simulink model "SWC_FDC_type"  (R2021b)
settings: Solver=FixedStepDiscrete  StartTime=0.0  StopTime=10.0  FixedStep=0.001  RelTol=1e-3
values from neighbouring files (symbols this model uses):
  DID_VCUKey = uint16(0x0202)    [vcu_local_hdr.m]
  DID_XWD = uint16(513)    [vcu_local_hdr.m]
  DIDLen_APSFunConfig = uint16(16)    [vcu_local_hdr.m]
  DIDLen_AutoLock = uint16(1)    [vcu_local_hdr.m]
  DIDLen_DKCKey = uint16(8)    [vcu_local_hdr.m]
  DIDLen_DRLDis = uint16(1)    [vcu_local_hdr.m]
  DIDLen_DynoMode = uint16(1)    [vcu_local_hdr.m]
  DIDLen_FMHTimer = uint16(1)    [vcu_local_hdr.m]
  DIDLen_LFLowPresThre = uint16(1)    [vcu_local_hdr.m]
  DIDLen_LFSensorID = uint16(4)    [vcu_local_hdr.m]
  DIDLen_LRLowPresThre = uint16(1)    [vcu_local_hdr.m]
  DIDLen_LRSensorID = uint16(4)    [vcu_local_hdr.m]
  DIDLen_RFLowPresThre = uint16(1)    [vcu_local_hdr.m]
  DIDLen_RFSensorID = uint16(4)    [vcu_local_hdr.m]
  DIDLen_RRLowPresThre = uint16(1)    [vcu_local_hdr.m]
  DIDLen_RRSensorID = uint16(4)    [vcu_local_hdr.m]
  DIDLen_SensorMode = uint16(1)    [vcu_local_hdr.m]
  DIDLen_TireSize = uint16(16)    [vcu_local_hdr.m]
  DIDLen_TPMSLearnSta = uint16(1)    [vcu_local_hdr.m]
  DIDLen_TurnLampFLThreCurr = uint16(1)    [vcu_local_hdr.m]
  DIDLen_TurnLampFRThreCurr = uint16(1)    [vcu_local_hdr.m]
  DIDLen_TurnLampRLThreCurr = uint16(1)    [vcu_local_hdr.m]
  DIDLen_TurnLampRRThreCurr = uint16(1)    [vcu_local_hdr.m]
  DIDLen_USSConfig = uint16(16)    [vcu_local_hdr.m]
  DIDLen_WhlPres = uint16(4)    [vcu_local_hdr.m]
  DIDLen_WhlSensorBattSta = uint16(1)    [vcu_local_hdr.m]
  DIDLen_WhlTmp = uint16(4)    [vcu_local_hdr.m]
  DIDLen_XWDMode = uint16(1)    [vcu_local_hdr.m]
  DIDNum_APSFunConfig = uint16(0x0903)    [vcu_local_hdr.m]
  DIDNum_AutoLock = uint16(0x0306)    [vcu_local_hdr.m]
  DIDNum_DKCKey = uint16(0x0202)    [vcu_local_hdr.m]
  DIDNum_DRLDis = uint16(0x0307)    [vcu_local_hdr.m]
  DIDNum_DynoMode = uint16(0x0203)    [vcu_local_hdr.m]
  DIDNum_FMHTimer = uint16(0x0305)    [vcu_local_hdr.m]
  DIDNum_LFLowPresThre = uint16(0x0B08)    [vcu_local_hdr.m]
  DIDNum_LFSensorID = uint16(0x0B01)    [vcu_local_hdr.m]
  DIDNum_LRLowPresThre = uint16(0x0B0A)    [vcu_local_hdr.m]
  DIDNum_LRSensorID = uint16(0x0B03)    [vcu_local_hdr.m]
  DIDNum_RFLowPresThre = uint16(0x0B09)    [vcu_local_hdr.m]
  DIDNum_RFSensorID = uint16(0x0B02)    [vcu_local_hdr.m]
  DIDNum_RRLowPresThre = uint16(0x0B0B)    [vcu_local_hdr.m]
  DIDNum_RRSensorID = uint16(0x0B04)    [vcu_local_hdr.m]
  DIDNum_SensorMode = uint16(0x0B0C)    [vcu_local_hdr.m]
  DIDNum_TireSize = uint16(0x0902)    [vcu_local_hdr.m]
  DIDNum_TPMSLearnSta = uint16(0x0B0D)    [vcu_local_hdr.m]
  DIDNum_TurnLampFLThreCurr = uint16(0x0303)    [vcu_local_hdr.m]
  DIDNum_TurnLampFRThreCurr = uint16(0x0301)    [vcu_local_hdr.m]
  DIDNum_TurnLampRLThreCurr = uint16(0x0304)    [vcu_local_hdr.m]
  DIDNum_TurnLampRRThreCurr = uint16(0x0302)    [vcu_local_hdr.m]
  DIDNum_USSConfig = uint16(0x0901)    [vcu_local_hdr.m]
  DIDNum_WhlPres = uint16(0x0B05)    [vcu_local_hdr.m]
  DIDNum_WhlSensorBattSta = uint16(0x0B07)    [vcu_local_hdr.m]
  DIDNum_WhlTmp = uint16(0x0B06)    [vcu_local_hdr.m]
  DIDNum_XWDMode = uint16(0x0201)    [vcu_local_hdr.m]
  DIDVCUKeyLength = uint16(8)    [vcu_local_hdr.m]
  ENUM_DRIVETRAIN_AWD = uint8(  2  )    [vcu_local_hdr.m]
  ENUM_DRIVETRAIN_FWD = uint8(  1  )    [vcu_local_hdr.m]
  ENUM_DRIVETRAIN_RWD = uint8(  0  )    [vcu_local_hdr.m]
  ENUM_REGENLEVEL_INVALID = uint8(  7  )    [vcu_local_hdr.m]
  ENUM_REGENLEVEL_LV1 = uint8(  1  )    [vcu_local_hdr.m]
  ENUM_REGENLEVEL_LV2 = uint8(  2  )    [vcu_local_hdr.m]
  ENUM_REGENLEVEL_LV3 = uint8(  3  )    [vcu_local_hdr.m]
  ENUM_REGENLEVEL_LV4 = uint8(  4  )    [vcu_local_hdr.m]
  ENUM_REGENLEVEL_LV5 = uint8(  5  )    [vcu_local_hdr.m]
  ENUM_REGENLEVEL_OFF = uint8(  0  )    [vcu_local_hdr.m]
  ENUM_REGENLEVEL_OPD = uint8(  6  )    [vcu_local_hdr.m]
  ENUM_TPMSLearnStatus_LEARNED = uint8(  1  )    [vcu_local_hdr.m]
  ENUM_TPMSLearnStatus_LEARNFAIL = uint8(  2  )    [vcu_local_hdr.m]
  ENUM_TPMSLearnStatus_NOTLEARN = uint8(  0  )    [vcu_local_hdr.m]
  ENUM_TPMSSTA_FAT = uint8(  8  )    [vcu_local_hdr.m]
  ENUM_TPMSSTA_LOWBATTERY = uint8(  2  )    [vcu_local_hdr.m]
  FALSE = boolean( 0 )    [vcu_local_hdr.m]
  ONE_INT = uint8(1)    [vcu_local_hdr.m]
  P_boolean = 0.0    [APPTypes.sldd]
  TRUE = boolean( 1 )    [vcu_local_hdr.m]
  ZERO_FLOAT = single(0)    [vcu_local_hdr.m]
  ZERO_INT = uint8(0)    [vcu_local_hdr.m]
undefined symbols (not defined in the file or in its folder): f32_ApsOutVehSpdSig, KHAL_DKCDecryptEnable_flg_ovrdflg, KHAL_DKCDecryptEnable_flg_ovrdval, KHAL_RandomNumberY1_enum, KHAL_RandomNumberY2_enum, KHAL_RandomNumberY_ovrdflg, KHAL_THCMAPTCWarningDTC_flg_ovrdflg, KHAL_THCMAPTCWarningDTC_flg_ovrdval, KHAL_TPMSRESBUTT_flg_ovrdflg, KHAL_TPMSRESBUTT_flg_ovrdval, R_DIDWriteCDD_CSOP_DIDSet_APSFunConfig, R_DIDWriteCDD_CSOP_DIDSet_AutoLock, R_DIDWriteCDD_CSOP_DIDSet_DKCKey, R_DIDWriteCDD_CSOP_DIDSet_DRLDis, R_DIDWriteCDD_CSOP_DIDSet_DynoMode, R_DIDWriteCDD_CSOP_DIDSet_FMHTimer, R_DIDWriteCDD_CSOP_DIDSet_LFLowPresThre, R_DIDWriteCDD_CSOP_DIDSet_LFSensorID, R_DIDWriteCDD_CSOP_DIDSet_LRLowPresThre, R_DIDWriteCDD_CSOP_DIDSet_LRSensorID, R_DIDWriteCDD_CSOP_DIDSet_RFLowPresThre, R_DIDWriteCDD_CSOP_DIDSet_RFSensorID, R_DIDWriteCDD_CSOP_DIDSet_RRLowPresThre, R_DIDWriteCDD_CSOP_DIDSet_RRSensorID, R_DIDWriteCDD_CSOP_DIDSet_SensorMode, R_DIDWriteCDD_CSOP_DIDSet_TireSize, R_DIDWriteCDD_CSOP_DIDSet_TPMSLearnSta, R_DIDWriteCDD_CSOP_DIDSet_TurnLampFLThreCurr, R_DIDWriteCDD_CSOP_DIDSet_TurnLampFRThreCurr, R_DIDWriteCDD_CSOP_DIDSet_TurnLampRLThreCurr, R_DIDWriteCDD_CSOP_DIDSet_TurnLampRRThreCurr, R_DIDWriteCDD_CSOP_DIDSet_USSConfig, R_DIDWriteCDD_CSOP_DIDSet_WhlPres, R_DIDWriteCDD_CSOP_DIDSet_WhlSensorBattSta, R_DIDWriteCDD_CSOP_DIDSet_WhlTmp, R_DIDWriteCDD_CSOP_DIDSet_XWDMode, R_E2E_CAN3_VCU1_CSOP_Write_CAN3_VCU1, R_E2E_CAN3_VCU1_toNIDEC_CSOP_Write_CAN3_VCU1_toNIDEC, R_E2E_CAN4_VCU1_CSOP_Write_CAN4_VCU1, R_FDCCDD_Inner_CSOP_FDC_AppCallSleep, R_HALINCDD_CSOP_PAS_Handler, R_HALINCDD_CSOP_UDS_Main, R_HALOUT_APS_CSOP_ApsOutput, R_HALOUTCDD_CSOP_AppNmStateReq, R_HALOUTCDD_CSOP_SetAcoreRebootCmdACK, R_HALOUTCDD_CSOP_SetSysPwrStat, R_HALOUTCDD_CSOP_SleepRequest, R_IOExpOUT_CDD_CSOP_IOExpSetVal, R_NVMReadCDD_Inner_NVM_ReadOperation, R_NVMWriteCDD_Inner_NVM_WriteOperation, R_UDSCDD_CSOP_DdmRestartOperationCycle, R_WDGCDD_CSOP_Call_Watchdog, R_WDGCDD_CSOP_Call_WDG_AppEnd, R_WDGCDD_CSOP_Call_WDG_AppStart, u16_DIDLen_APSFunConfig, u16_DIDLen_AutoLock, u16_DIDLen_DKCKey, u16_DIDLen_DRLDis, u16_DIDLen_DynoMode, u16_DIDLen_FMHTimer ... (+83)
libraries: simulink x215, FVT_lib x139, hcu_lib x21, hdlsllib x9, app x1, halin x1, halout x1, inp x1, outp x1
(part 9 of 12)

== system SWC_FDC_type/run_SWC_FDC_RxTx_5ms_sys/OUTP_AFTER/Subsystem5 ==
  BOUTP_outputs : Inport
  BHAL_SYSTPMS_outputs : Inport  Port=2
  BHAL_SYS_outputs : Inport  Port=3
  Bus Selector : BusSelector  OutputSignals=VOUTP_AntitheftSta_enum,VOUTP_DrivetrainSelect_enum,VOUTP_WriteChkLFID_raw,VOUTP_WriteChkRFID_raw,VOUTP_WriteChkLRID_raw,VOUTP_WriteChkRRID_raw,VOUTP_WriteChkfinLFID_raw,VOUTP_WriteChkfinRFID_raw,VOUTP_WriteChkfinLRID_raw,VOUTP_WriteChkfinRRID_raw,VOUTP_LFSensorFail_flg,VOUTP_RFSensorFail_flg,VOUTP_LRSensorFail_flg,VOUTP_RRSensorFail_flg,VOUTP_LFWheelPSW_raw8,VOUTP_RFWheelPSW_raw8,VOUTP_LRWheelPSW_raw8,VOUTP_RRWheelPSW_raw8,VOUTP_LFPindi_enum,VOUTP_RFPind_enum,VOUTP_LRPindi_enum,VOUTP_RRPindi_enum,VOUTP_LFP20_raw8,VOUTP_RFP20_raw8,VOUTP_LRP20_raw8,VOUTP_RRP20_raw8,VOUTP_LFWheelPress_raw8,VOUTP_RFWheelPress_raw8,VOUTP_LRWheelPress_raw8,VOUTP_RRWheelPress_raw8,VOUTP_LFWheelTemp_C,VOUTP_RFWheelTemp_C,VOUTP_LRWheelTemp_C,VOUTP_RRWheelTemp_C,VOUTP_Flashchkdatavalid_enum,VOUTP_Flashdatavalid_enum,VOUTP_unlearnSfali_flg,VOUTP_unlearnSfailvalid_enum,VOUTP_Prepresstempvalid_enum,VOUTP_FlashS1ID_raw,VOUTP_FlashS2ID_raw,VOUTP_FlashS3ID_raw,VOUTP_FlashS4ID_raw,VOUTP_FlashIDvalid_enum,VOUTP_ACModeMem_enum,VOUTP_Face_flg,VOUTP_Foot_flg,VOUTP_Frost_flg,VOUTP_FaceM_flg,VOUTP_FootM_flg,VOUTP_CCUSyncSts_flg,VOUTP_ACForceOFF_flg,VOUTP_sigRecircSt_flg,VOUTP_RecAutoFlg_flg,VOUTP_AirIntenZone1M_enum,VOUTP_fdefog_flg,VOUTP_sigSetTempZon1St_C,VOUTP_sigSetTempZon2StM_C,VOUTP_CountAlarm_enum,VOUTP_MFSWTri_flg,VOUTP_MirrorFlodPos_flg,VOUTP_FuelDoorPos_flg,VOUTP_LockSetting_flg,VOUTP_MFRDNBrightReq_pct,VOUTP_RoomLampMode_flg,VOUTP_WiperFixMode_flg,VOUTP_IVIPTGUSStaSW_flg,VOUTP_EAPS1MIN_pct,VOUTP_EAPS2MIN_pct,VOUTP_HoodSW_flg,VOUTP_TailgateSW_flg,VOUTP_CTDLockSW_flg,VOUTP_TailgateHDSW_flg,VOUTP_APMDoorControlSta_flg,VOUTP_fUnlockSingle_flg,VOUTP_SaveRegenMode_enum,VOUTP_AmbFunENFlash_enum,VOUTP_AmbWelENFlash_enum,VOUTP_AmbDimENFlash_enum,VOUTP_AmbLinkDriStaFlash_enum,VOUTP_AmbPwrWarnENFlash_enum,VOUTP_AmbODAENFlash_enum,VOUTP_AmbColorSta1_enum,VOUTP_AmbColorSta2_enum,VOUTP_AmbColorSta3_enum,VOUTP_AmbColorSta4_enum,VOUTP_AmbColorSta5_enum,VOUTP_AmbColorSta7_enum,VOUTP_AmbBrightnessSta1_enum,VOUTP_AmbBrightnessSta2_enum,VOUTP_AmbBrightnessSta3_enum,VOUTP_AmbBrightnessSta4_enum,VOUTP_AmbBrightnessSta5_enum,VOUTP_AmbBrightnessSta7_enum
  Bus Selector1 : BusSelector  OutputSignals=VHAL_RandomnumberY_raw1,VHAL_RandomnumberY_raw2,VHAL_RandomnumberY_raw3,VHAL_RandomnumberY_raw4,VHAL_RandomnumberY_raw5,VHAL_RandomnumberY_raw6,VHAL_RandomnumberY_raw7,VHAL_RandomnumberY_raw8,VHAL_funAuto_flg,VHAL_DiagDRLOFF_flg,VHAL_DiagFMHT_s,VHAL_DiagFLTC_mA,VHAL_DiagFRTC_mA,VHAL_DiagRLTC_mA,VHAL_DiagRRTC_mA,VHAL_USSConfig_raw8,VHAL_TireSize_raw8,VHAL_APSFunConfig_raw8
  Enabled Subsystem : Subsystem  TreatAsAtomicUnit=on
  HAL_NvmWriteData_raw : Outport
  wires:
  BOUTP_outputs/1 -> Bus Selector/1
  Enabled Subsystem/1(HAL_NvmWriteData_raw) -> HAL_NvmWriteData_raw/1
  Bus Selector1/2 -> Enabled Subsystem/97(VHAL_RandomnumberY_raw2)  "<VHAL_RandomnumberY_raw2>"
  Bus Selector1/3 -> Enabled Subsystem/98(VHAL_RandomnumberY_raw3)  "<VHAL_RandomnumberY_raw3>"
  Bus Selector1/4 -> Enabled Subsystem/99(VHAL_RandomnumberY_raw4)  "<VHAL_RandomnumberY_raw4>"
  Bus Selector1/5 -> Enabled Subsystem/100(VHAL_RandomnumberY_raw5)  "<VHAL_RandomnumberY_raw5>"
  Bus Selector1/6 -> Enabled Subsystem/101(VHAL_RandomnumberY_raw6)  "<VHAL_RandomnumberY_raw6>"
  Bus Selector1/7 -> Enabled Subsystem/102(VHAL_RandomnumberY_raw7)  "<VHAL_RandomnumberY_raw7>"
  Bus Selector1/8 -> Enabled Subsystem/103(VHAL_RandomnumberY_raw8)  "<VHAL_RandomnumberY_raw8>"
  Bus Selector/24 -> Enabled Subsystem/24(VOUTP_RFP20_raw8)  "<VOUTP_RFP20_raw8>"
  Bus Selector/23 -> Enabled Subsystem/23(VOUTP_LFP20_raw8)  "<VOUTP_LFP20_raw8>"
  Bus Selector/25 -> Enabled Subsystem/25(VOUTP_LRP20_raw8)  "<VOUTP_LRP20_raw8>"
  Bus Selector/22 -> Enabled Subsystem/22(VOUTP_RRPindi_enum)  "<VOUTP_RRPindi_enum>"
  Bus Selector/26 -> Enabled Subsystem/26(VOUTP_RRP20_raw8)  "<VOUTP_RRP20_raw8>"
  Bus Selector/21 -> Enabled Subsystem/21(VOUTP_LRPindi_enum)  "<VOUTP_LRPindi_enum>"
  Bus Selector/27 -> Enabled Subsystem/27(VOUTP_LFWheelPress_raw8)  "<VOUTP_LFWheelPress_raw8>"
  Bus Selector/20 -> Enabled Subsystem/20(VOUTP_RFPindi_enum)  "<VOUTP_RFPind_enum>"
  Bus Selector/28 -> Enabled Subsystem/28(VOUTP_RFWheelPress_raw8)  "<VOUTP_RFWheelPress_raw8>"
  Bus Selector/19 -> Enabled Subsystem/19(VOUTP_LFPindi_enum)  "<VOUTP_LFPindi_enum>"
  Bus Selector/29 -> Enabled Subsystem/29(VOUTP_LRWheelPress_raw8)  "<VOUTP_LRWheelPress_raw8>"
  Bus Selector/56 -> Enabled Subsystem/56(VOUTP_fdefog_flg)  "<VOUTP_fdefog_flg>"
  Bus Selector/18 -> Enabled Subsystem/18(VOUTP_RRWheelPSW_raw8)  "<VOUTP_RRWheelPSW_raw8>"
  Bus Selector/30 -> Enabled Subsystem/30(VOUTP_RRWheelPress_raw8)  "<VOUTP_RRWheelPress_raw8>"
  Bus Selector/55 -> Enabled Subsystem/55(VOUTP_AirIntenZone1M_enum)  "<VOUTP_AirIntenZone1M_enum>"
  Bus Selector/17 -> Enabled Subsystem/17(VOUTP_LRWheelPSW_raw8)  "<VOUTP_LRWheelPSW_raw8>"
  Bus Selector/31 -> Enabled Subsystem/31(VOUTP_LFWheelTemp_C)  "<VOUTP_LFWheelTemp_C>"
  Bus Selector/54 -> Enabled Subsystem/54(VOUTP_RecAutoFlg_flg)  "<VOUTP_RecAutoFlg_flg>"
  Bus Selector/16 -> Enabled Subsystem/16(VOUTP_RFWheelPSW_raw8)  "<VOUTP_RFWheelPSW_raw8>"
  Bus Selector/32 -> Enabled Subsystem/32(VOUTP_RFWheelTemp_C)  "<VOUTP_RFWheelTemp_C>"
  Bus Selector/53 -> Enabled Subsystem/53(VOUTP_sigRecircSt_flg)  "<VOUTP_sigRecircSt_flg>"
  Bus Selector/15 -> Enabled Subsystem/15(VOUTP_LFWheelPSW_raw8)  "<VOUTP_LFWheelPSW_raw8>"
  Bus Selector/33 -> Enabled Subsystem/33(VOUTP_LRWheelTemp_C)  "<VOUTP_LRWheelTemp_C>"
  Bus Selector/52 -> Enabled Subsystem/52(VOUTP_ACForceOFF_flg)  "<VOUTP_ACForceOFF_flg>"
  Bus Selector/14 -> Enabled Subsystem/14(VOUTP_RRSensorFail_flg)  "<VOUTP_RRSensorFail_flg>"
  Bus Selector/34 -> Enabled Subsystem/34(VOUTP_RRWheelTemp_C)  "<VOUTP_RRWheelTemp_C>"
  Bus Selector/51 -> Enabled Subsystem/51(VOUTP_CCUSyncSts_flg)  "<VOUTP_CCUSyncSts_flg>"
  Bus Selector/13 -> Enabled Subsystem/13(VOUTP_LRSensorFail_flg)  "<VOUTP_LRSensorFail_flg>"
  Bus Selector/35 -> Enabled Subsystem/35(VOUTP_Flashchkdatavalid_enum)  "<VOUTP_Flashchkdatavalid_enum>"
  Bus Selector/50 -> Enabled Subsystem/50(VOUTP_FootM_flg)  "<VOUTP_FootM_flg>"
  Bus Selector/12 -> Enabled Subsystem/12(VOUTP_RFSensorFail_flg)  "<VOUTP_RFSensorFail_flg>"
  Bus Selector/36 -> Enabled Subsystem/36(VOUTP_Flashdatavalid_enum)  "<VOUTP_Flashdatavalid_enum>"
  Bus Selector/49 -> Enabled Subsystem/49(VOUTP_FaceM_flg)  "<VOUTP_FaceM_flg>"
  Bus Selector/11 -> Enabled Subsystem/11(VOUTP_LFSensorFail_flg)  "<VOUTP_LFSensorFail_flg>"
  Bus Selector/37 -> Enabled Subsystem/37(VOUTP_unlearnSfali_flg)  "<VOUTP_unlearnSfali_flg>"
  Bus Selector/48 -> Enabled Subsystem/48(VOUTP_Frost_flg)  "<VOUTP_Frost_flg>"
  Bus Selector/38 -> Enabled Subsystem/38(VOUTP_unlearnSfailvalid_enum)  "<VOUTP_unlearnSfailvalid_enum>"
  Bus Selector/47 -> Enabled Subsystem/47(VOUTP_Foot_flg)  "<VOUTP_Foot_flg>"
  Bus Selector/39 -> Enabled Subsystem/39(VOUTP_Prepresstempvalid_enum)  "<VOUTP_Prepresstempvalid_enum>"
  Bus Selector/46 -> Enabled Subsystem/46(VOUTP_Face_flg)  "<VOUTP_Face_flg>"
  Bus Selector/2 -> Enabled Subsystem/2(VOUTP_DrivetrainSelect_enum)  "<VOUTP_DrivetrainSelect_enum>"
  Bus Selector/1 -> Enabled Subsystem/1(VOUTP_AntitheftSta_enum)  "<VOUTP_AntitheftSta_enum>"
  BHAL_SYSTPMS_outputs/1 -> Enabled Subsystem/95(BHAL_SYSTPMS_outputs)
  Bus Selector/10 -> Enabled Subsystem/10(VOUTP_WriteChkfinRRID_raw)  "<VOUTP_WriteChkfinRRID_raw>"
  Bus Selector/9 -> Enabled Subsystem/9(VOUTP_WriteChkfinLRID_raw)  "<VOUTP_WriteChkfinLRID_raw>"
  Bus Selector/8 -> Enabled Subsystem/8(VOUTP_WriteChkfinRFID_raw)  "<VOUTP_WriteChkfinRFID_raw>"
  Bus Selector/7 -> Enabled Subsystem/7(VOUTP_WriteChkfinLFID_raw)  "<VOUTP_WriteChkfinLFID_raw>"
  Bus Selector/6 -> Enabled Subsystem/6(VOUTP_WriteChkRRID_raw)  "<VOUTP_WriteChkRRID_raw>"
  Bus Selector/5 -> Enabled Subsystem/5(VOUTP_WriteChkLRID_raw)  "<VOUTP_WriteChkLRID_raw>"
  Bus Selector/4 -> Enabled Subsystem/4(VOUTP_WriteChkRFID_raw)  "<VOUTP_WriteChkRFID_raw>"
  Bus Selector/3 -> Enabled Subsystem/3(VOUTP_WriteChkLFID_raw)  "<VOUTP_WriteChkLFID_raw>"
  Bus Selector/58 -> Enabled Subsystem/58(VOUTP_sigSetTempZon2StM_C)  "<VOUTP_sigSetTempZon2StM_C>"
  Bus Selector/59 -> Enabled Subsystem/59(VOUT_CountAlarm_enum)  "<VOUTP_CountAlarm_enum>"
  Bus Selector/57 -> Enabled Subsystem/57(VOUTP_sigSetTempZon1St_C)  "<VOUTP_sigSetTempZon1St_C>"
  Bus Selector/60 -> Enabled Subsystem/60(VOUTP_MFSWTri_flg)  "<VOUTP_MFSWTri_flg>"
  Bus Selector/61 -> Enabled Subsystem/61(VOUTP_MirrorFlodPos_flg)  "<VOUTP_MirrorFlodPos_flg>"
  Bus Selector/62 -> Enabled Subsystem/62(VOUTP_FuelDoorPos_flg)  "<VOUTP_FuelDoorPos_flg>"
  Bus Selector/63 -> Enabled Subsystem/63(VOUTP_LockSetting_flg)  "<VOUTP_LockSetting_flg>"
  Bus Selector/64 -> Enabled Subsystem/64(VOUTP_MFRDNBrightReq_pct)  "<VOUTP_MFRDNBrightReq_pct>"
  Bus Selector/65 -> Enabled Subsystem/65(VOUTP_RoomLampMode_flg)  "<VOUTP_RoomLampMode_flg>"
  Bus Selector/66 -> Enabled Subsystem/66(VOUTP_WiperFixMode_flg)  "<VOUTP_WiperFixMode_flg>"
  Bus Selector/67 -> Enabled Subsystem/67(VOUTP_IVIPTGUSStaSW_flg)  "<VOUTP_IVIPTGUSStaSW_flg>"
  Bus Selector1/1 -> Enabled Subsystem/96(VHAL_RandomnumberY_raw1)  "<VHAL_RandomnumberY_raw1>"
  Bus Selector/45 -> Enabled Subsystem/45(VOUTP_ACModeMem_enum)  "<VOUTP_ACModeMem_enum>"
  Bus Selector/40 -> Enabled Subsystem/40(VOUTP_FlashS1ID_raw)  "<VOUTP_FlashS1ID_raw>"
  Bus Selector/41 -> Enabled Subsystem/41(VOUTP_FlashS2ID_raw)  "<VOUTP_FlashS2ID_raw>"
  Bus Selector/42 -> Enabled Subsystem/42(VOUTP_FlashS3ID_raw)  "<VOUTP_FlashS3ID_raw>"
  Bus Selector/43 -> Enabled Subsystem/43(VOUTP_FlashS41ID_raw)  "<VOUTP_FlashS4ID_raw>"
  Bus Selector/44 -> Enabled Subsystem/44(VOUTP_FlashIDvalid_enum)  "<VOUTP_FlashIDvalid_enum>"
  BHAL_SYS_outputs/1 -> Bus Selector1/1
  Bus Selector/68 -> Enabled Subsystem/68(VOUTP_EAPS1MIN_pct)  "<VOUTP_EAPS1MIN_pct>"
  Bus Selector/69 -> Enabled Subsystem/69(VOUTP_EAPS2MIN_pct)  "<VOUTP_EAPS2MIN_pct>"
  Bus Selector/70 -> Enabled Subsystem/70(VOUTP_HoodSW_flg)  "<VOUTP_HoodSW_flg>"
  Bus Selector/71 -> Enabled Subsystem/71(VOUTP_TailgateSW_flg)  "<VOUTP_TailgateSW_flg>"
  Bus Selector/72 -> Enabled Subsystem/72(VOUTP_CTDLockSW_flg)  "<VOUTP_CTDLockSW_flg>"
  Bus Selector/73 -> Enabled Subsystem/73(VOUTP_TailgateHDSW_flg)  "<VOUTP_TailgateHDSW_flg>"
  Bus Selector/74 -> Enabled Subsystem/74(VOUTP_APMDoorControlSta_flg)  "<VOUTP_APMDoorControlSta_flg>"
  Bus Selector1/9 -> Enabled Subsystem/104(VHAL_funAuto_flg)  "<VHAL_funAuto_flg>"
  Bus Selector1/10 -> Enabled Subsystem/105(VHAL_DiagDRLOFF_flg)  "<VHAL_DiagDRLOFF_flg>"
  Bus Selector1/11 -> Enabled Subsystem/106(VHAL_DiagFMHT_s)  "<VHAL_DiagFMHT_s>"
  Bus Selector1/12 -> Enabled Subsystem/107(VHAL_DiagFLTC_mA)  "<VHAL_DiagFLTC_mA>"
  Bus Selector1/13 -> Enabled Subsystem/108(VHAL_DiagFRTC_mA)  "<VHAL_DiagFRTC_mA>"
  Bus Selector1/14 -> Enabled Subsystem/109(VHAL_DiagRLTC_mA)  "<VHAL_DiagRLTC_mA>"
  Bus Selector1/15 -> Enabled Subsystem/110(VHAL_DiagRRTC_mA)  "<VHAL_DiagRRTC_mA>"
  Bus Selector1/16 -> Enabled Subsystem/111(VHAL_USSConfig_raw8)  "<VHAL_USSConfig_raw8>"
  Bus Selector1/17 -> Enabled Subsystem/112(VHAL_TireSize_raw8)  "<VHAL_TireSize_raw8>"
  Bus Selector1/18 -> Enabled Subsystem/113(VHAL_APSFunConfig_raw8)  "<VHAL_APSFunConfig_raw8>"
  Bus Selector/75 -> Enabled Subsystem/75(VOUTP_fUnlockSingle_flg)  "<VOUTP_fUnlockSingle_flg>"
  Bus Selector/76 -> Enabled Subsystem/76(VOUTP_SaveRegenMode_enum)  "<VOUTP_SaveRegenMode_enum>"
  Bus Selector/77 -> Enabled Subsystem/77(VOUTP_AmbFunENFlash_enum)  "<VOUTP_AmbFunENFlash_enum>"
  Bus Selector/78 -> Enabled Subsystem/78(VOUTP_AmbWelENFlash_enum)  "<VOUTP_AmbWelENFlash_enum>"
  Bus Selector/79 -> Enabled Subsystem/79(VOUTP_AmbDimENFlash_enum)  "<VOUTP_AmbDimENFlash_enum>"
  Bus Selector/80 -> Enabled Subsystem/80(VOUTP_AmbLinkDriStaFlash_enum)  "<VOUTP_AmbLinkDriStaFlash_enum>"
  Bus Selector/81 -> Enabled Subsystem/81(VOUTP_AmbPwrWarnENFlash_enum)  "<VOUTP_AmbPwrWarnENFlash_enum>"
  Bus Selector/82 -> Enabled Subsystem/82(VOUTP_AmbODAENFlash_enum)  "<VOUTP_AmbODAENFlash_enum>"
  Bus Selector/83 -> Enabled Subsystem/83(VOUTP_AmbColorSta1_enum)  "<VOUTP_AmbColorSta1_enum>"
  Bus Selector/84 -> Enabled Subsystem/84(VOUTP_AmbColorSta2_enum)  "<VOUTP_AmbColorSta2_enum>"
  Bus Selector/85 -> Enabled Subsystem/85(VOUTP_AmbColorSta3_enum)  "<VOUTP_AmbColorSta3_enum>"
  Bus Selector/86 -> Enabled Subsystem/86(VOUTP_AmbColorSta4_enum)  "<VOUTP_AmbColorSta4_enum>"
  Bus Selector/87 -> Enabled Subsystem/87(VOUTP_AmbColorSta5_enum)  "<VOUTP_AmbColorSta5_enum>"
  Bus Selector/88 -> Enabled Subsystem/88(VOUTP_AmbColorSta7_enum)  "<VOUTP_AmbColorSta7_enum>"
  Bus Selector/89 -> Enabled Subsystem/89(VOUTP_AmbBrightnessSta1_enum)  "<VOUTP_AmbBrightnessSta1_enum>"
  Bus Selector/90 -> Enabled Subsystem/90(VOUTP_AmbBrightnessSta2_enum)  "<VOUTP_AmbBrightnessSta2_enum>"
  Bus Selector/91 -> Enabled Subsystem/91(VOUTP_AmbBrightnessSta3_enum)  "<VOUTP_AmbBrightnessSta3_enum>"
  Bus Selector/92 -> Enabled Subsystem/92(VOUTP_AmbBrightnessSta4_enum)  "<VOUTP_AmbBrightnessSta4_enum>"
  Bus Selector/93 -> Enabled Subsystem/93(VOUTP_AmbBrightnessSta5_enum)  "<VOUTP_AmbBrightnessSta5_enum>"
  Bus Selector/94 -> Enabled Subsystem/94(VOUTP_AmbBrightnessSta7_enum)  "<VOUTP_AmbBrightnessSta7_enum>"

== system SWC_FDC_type/run_SWC_FDC_RxTx_5ms_sys/Subsystem2/DKC2 ==
  Enable_Decrypt : Inport
  DKC_ResultData_16byte : Inport  Port=2
  BHAL_CAN4_outputs : Inport  Port=3
  Bus Creator1 : BusCreator  Inputs=14
  DKC Decryption and Unpack : Subsystem
  Data Type Conversion{1,41..51,53..54} (14 alike) : DataTypeConversion
  BHAL_DKC_outputs : Outport
  wires:
  DKC Decryption and Unpack/1(VHAL_DKCDecReVehData_enum) -> Data Type Conversion53/1
  DKC Decryption and Unpack/2(VHAL_DKCDecRemotePW_enum) -> Data Type Conversion54/1
  DKC Decryption and Unpack/3(VHAL_DKCDecPCommandToBCM_enum) -> Data Type Conversion41/1
  DKC Decryption and Unpack/4(VHAL_DKCDecPCommandToPTG_enum) -> Data Type Conversion42/1
  DKC Decryption and Unpack/5(VHAL_DKCDecPDKeyAreaLockUnlock_enum) -> Data Type Conversion43/1
  DKC Decryption and Unpack/6(VHAL_DKCDecPDKeyAreaPS_enum) -> Data Type Conversion44/1
  DKC Decryption and Unpack/7(VHAL_DKCDecPDKeyAreaPTG_enum) -> Data Type Conversion45/1
  DKC Decryption and Unpack/8(VHAL_DKCDecPDKeyWelcome_enum) -> Data Type Conversion49/1
  DKC Decryption and Unpack/13(VHAL_TimeSNDKCFbk_cnt) -> Data Type Conversion48/1
  DKC Decryption and Unpack/9(VHAL_DKCDecPDkeyShowIVI_enum) -> Data Type Conversion50/1
  DKC Decryption and Unpack/12(VHAL_DKCDecPUIDLowPower_flg) -> Data Type Conversion47/1
  DKC Decryption and Unpack/10(VHAL_DKCDecPKeyMiss_flg) -> Data Type Conversion51/1
  DKC Decryption and Unpack/11(VHAL_DKCDecPKeyMode_enum) -> Data Type Conversion46/1
  Data Type Conversion43/1 -> Bus Creator1/5  "VHAL_DKCDecPDKeyAreaLockUnlock_enum"
  Data Type Conversion54/1 -> Bus Creator1/2  "VHAL_DKCDecRemotePW_enum"
  Data Type Conversion53/1 -> Bus Creator1/1  "VHAL_DKCDecReVehData_enum"
  Data Type Conversion41/1 -> Bus Creator1/3  "VHAL_DKCDecPCommandToBCM_enum"
  Data Type Conversion46/1 -> Bus Creator1/11  "VHAL_DKCDecPKeyMode_enum"
  Data Type Conversion47/1 -> Bus Creator1/12  "VHAL_DKCDecPUIDLowPower_flg"
  Data Type Conversion42/1 -> Bus Creator1/4  "VHAL_DKCDecPCommandToPTG_enum"
  Data Type Conversion50/1 -> Bus Creator1/9  "VHAL_DKCDecPDkeyShowIVI_enum"
  Bus Creator1/1 -> BHAL_DKC_outputs/1  "BHAL_DKC_outputs"
  Data Type Conversion51/1 -> Bus Creator1/10  "VHAL_DKCDecPKeyMiss_flg"
  Data Type Conversion49/1 -> Bus Creator1/8  "VHAL_DKCDecPDKeyWelcome_enum"
  Data Type Conversion48/1 -> Bus Creator1/13  "VHAL_TimeSNDKCFbk_cnt"
  Data Type Conversion45/1 -> Bus Creator1/7  "VHAL_DKCDecPDKeyAreaPTG_enum"
  Data Type Conversion44/1 -> Bus Creator1/6  "VHAL_DKCDecPDKeyAreaPS_enum"
  DKC_ResultData_16byte/1 -> DKC Decryption and Unpack/1(DKC_ResultData_16byte)
  DKC Decryption and Unpack/14(VHAL_DKCDecryptionFail_flg) -> Data Type Conversion1/1
  Data Type Conversion1/1 -> Bus Creator1/14  "VHAL_DKCDecryptionFail_flg"
  BHAL_CAN4_outputs/1 -> DKC Decryption and Unpack/2(BHAL_CAN4_outputs)
  Enable_Decrypt/1 -> DKC Decryption and Unpack/Enable

== system SWC_FDC_type/run_SWC_FDC_RxTx_5ms_sys/Halin_CDD/Halin_APM/Subsystem ==
  PASDistanceData : Inport
  APSDistanceData : Inport  Port=2
  APSLevelData : Inport  Port=3
  APSFaultStaData : Inport  Port=4
  ChimeIn : Inport  Port=5
  SNSRLayoutIn : Inport  Port=6
  StaFSyaIn : Inport  Port=7
  ModOperationIn : Inport  Port=8
  Demux : Demux  Outputs=8
  Demux1 : Demux  Outputs=12
  Demux2 : Demux  Outputs=8
  Demux3 : Demux
  PASDFCR : Outport
  PASDFMR : Outport  Port=2
  PASDFML : Outport  Port=3
  PASDFCL : Outport  Port=4
  PASDRCR : Outport  Port=5
  PASDRMR : Outport  Port=6
  PASDRML : Outport  Port=7
  PASDRCL : Outport  Port=8
  APSDFLL : Outport  Port=9
  APSDRLL : Outport  Port=10
  APSDFLR : Outport  Port=11
  APSDRLR : Outport  Port=12
  PASAFCR : Outport  Port=13
  PASAFMR : Outport  Port=14
  PASAFML : Outport  Port=15
  PASAFCL : Outport  Port=16
  PASARCR : Outport  Port=17
  PASARMR : Outport  Port=18
  PASARML : Outport  Port=19
  PASARCL : Outport  Port=20
  USSStaFCR : Outport  Port=21
  USSStaFMR : Outport  Port=22
  USSStaFML : Outport  Port=23
  USSStaFCL : Outport  Port=24
  USSStaRCR : Outport  Port=25
  USSStaRMR : Outport  Port=26
  USSStaRML : Outport  Port=27
  USSStaRCL : Outport  Port=28
  USSStaFLL : Outport  Port=29
  USSStaRLL : Outport  Port=30
  USSStaFLR : Outport  Port=31
  USSStaRLR : Outport  Port=32
  Chime : Outport  Port=33
  SNSRLayout : Outport  Port=34
  StaFSya : Outport  Port=35
  ModOperation : Outport  Port=36
  wires:
  Demux/8 -> [PASDRCL]
  Demux/7 -> [PASDRML]
  Demux/6 -> [PASDRMR]
  Demux/5 -> [PASDRCR]
  Demux/4 -> [PASDFCL]
  Demux/3 -> [PASDFML]
  Demux/2 -> [PASDFMR]
  Demux/1 -> [PASDFCR]
  [PASDRML] -> PASDRML/1
  [PASDRLR] -> APSDRLR/1
  [PASDFMR] -> PASDFMR/1
  [PASDFCL] -> PASDFCL/1
  [PASDRCL] -> PASDRCL/1
  [PASDRMR] -> PASDRMR/1
  [PASDRCR] -> PASDRCR/1
  [PASDFLL] -> APSDFLL/1
  [PASDFLR] -> APSDFLR/1
  [PASDRLL] -> APSDRLL/1
  [PASDFML] -> PASDFML/1
  Demux1/1 -> [USSStaFCR]
  ModOperationIn/1 -> ModOperation/1
  SNSRLayoutIn/1 -> SNSRLayout/1
  [PASDistanceData] -> Demux/1
  [PASDFCR] -> PASDFCR/1
  ChimeIn/1 -> Chime/1
  Demux1/2 -> [USSStaFMR]
  StaFSyaIn/1 -> StaFSya/1
  [APSFaultStaData] -> Demux1/1
  [APSLevelData] -> Demux2/1
  Demux2/1 -> [PASAFCR]
  Demux2/2 -> [PASAFMR]
  Demux2/3 -> [PASAFML]
  Demux2/4 -> [PASAFCL]
  Demux2/5 -> [PASARCR]
  Demux2/6 -> [PASARMR]
  Demux2/7 -> [PASARML]
  Demux2/8 -> [PASARCL]
  [PASAFCR] -> PASAFCR/1
  [PASAFMR] -> PASAFMR/1
  [PASAFML] -> PASAFML/1
  [PASAFCL] -> PASAFCL/1
  [PASARCR] -> PASARCR/1
  [PASARMR] -> PASARMR/1
  [PASARML] -> PASARML/1
  [PASARCL] -> PASARCL/1
  Demux1/3 -> [USSStaFML]
  Demux1/4 -> [USSStaFCL]
  Demux1/6 -> [USSStaRMR]
  Demux1/7 -> [USSStaRML]
  Demux1/9 -> [USSStaFLL]
  Demux1/10 -> [USSStaRLL]
  Demux1/12 -> [USSStaRLR]
  Demux1/11 -> [USSStaFLR]
  Demux1/5 -> [USSStaRCR]
  Demux1/8 -> [USSStaRCL]
  [USSStaFCR] -> USSStaFCR/1
  [USSStaFMR] -> USSStaFMR/1
  [USSStaFML] -> USSStaFML/1
  [USSStaFCL] -> USSStaFCL/1
  [USSStaRCR] -> USSStaRCR/1
  [USSStaRMR] -> USSStaRMR/1
  [USSStaRML] -> USSStaRML/1
  [USSStaRCL] -> USSStaRCL/1
  [USSStaFLL] -> USSStaFLL/1
  [USSStaRLL] -> USSStaRLL/1
  [USSStaFLR] -> USSStaFLR/1
  [USSStaRLR] -> USSStaRLR/1
  APSDistanceData/1 -> [APSDistanceData]
  APSLevelData/1 -> [APSLevelData]
  APSFaultStaData/1 -> [APSFaultStaData]
  PASDistanceData/1 -> [PASDistanceData]
  [APSDistanceData] -> Demux3/1
  Demux3/1 -> [PASDFLL]
  Demux3/2 -> [PASDRLL]
  Demux3/3 -> [PASDFLR]
  Demux3/4 -> [PASDRLR]

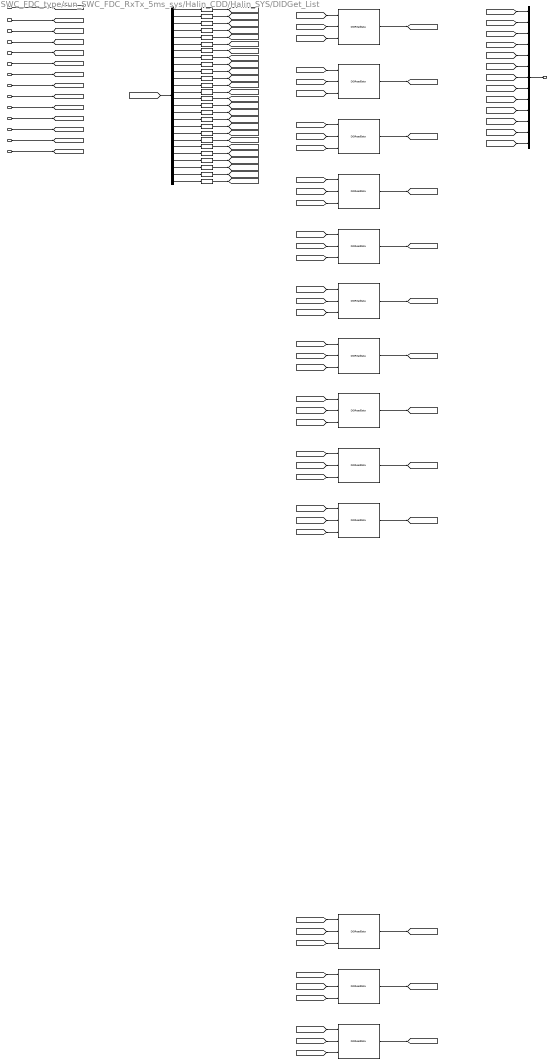
== system SWC_FDC_type/run_SWC_FDC_RxTx_5ms_sys/Halin_CDD/Halin_SYS/DIDGet_List ==
  BHAL_DIDGetData_raw : Inport
  VHAL_DIDFlashXWDMode_raw8 : Inport  Port=2
  VHAL_DIDFlashDKCKey_raw8 : Inport  Port=3
  VHAL_DIDFlashDynoMode_raw8 : Inport  Port=4
  VHAL_DIDFlashTurnLampFRThreCurr_raw8 : Inport  Port=5
  VHAL_DIDFlashTurnLampRRThreCurr_raw8 : Inport  Port=6
  VHAL_DIDFlashTurnLampFLThreCurr_raw8 : Inport  Port=7
  VHAL_DIDFlashTurnLampRLThreCurr_raw8 : Inport  Port=8
  VHAL_DIDFlashFMHTimer_raw8 : Inport  Port=9
  VHAL_DIDFlashAutoLock_raw8 : Inport  Port=10
  VHAL_DIDFlashDRLDis_raw8 : Inport  Port=11
  VHAL_DIDFlashUSSConfig_raw8 : Inport  Port=12
  VHAL_DIDFlashTireSize_raw8 : Inport  Port=13
  VHAL_DIDFlashAPSFunConfig_raw8 : Inport  Port=14
  AutoLock : hcu_lib/Basic_Blocks/DIDReadData
  DRLDisable : hcu_lib/Basic_Blocks/DIDReadData
  Dyno mode switch : hcu_lib/Basic_Blocks/DIDReadData
  FollowMeHomeTimer : hcu_lib/Basic_Blocks/DIDReadData
  TurnLampFrontLeftThresholdCurrent : hcu_lib/Basic_Blocks/DIDReadData
  TurnLampFrontRightThresholdCurrent : hcu_lib/Basic_Blocks/DIDReadData
  TurnLampRearLeftThresholdCurrent : hcu_lib/Basic_Blocks/DIDReadData
  TurnLampRearRightThresholdCurrent : hcu_lib/Basic_Blocks/DIDReadData
  UnitConverter{,1..25} (26 alike) : DataTypeConversion  OutDataTypeStr=uint8
  WriteRandomNumberDKC : hcu_lib/Basic_Blocks/DIDReadData
  XWD switch : hcu_lib/Basic_Blocks/DIDReadData
  apsFunctionConfiguration : hcu_lib/Basic_Blocks/DIDReadData
  apsUssConfiguration : hcu_lib/Basic_Blocks/DIDReadData
  apsVehicleTireSize : hcu_lib/Basic_Blocks/DIDReadData
  bus_Creator : BusCreator  Inputs=13
  bus_selector : BusSelector  OutputSignals=u8_DIDSta_XWDMode,u8_XWDMode,u8_DIDSta_DKCKey,u8Array8_DKCKey,u8_DIDSta_DynoMode,u8_DynoMode,u8_DIDSta_TurnLampFRThreCurr,u8_TurnLampFRThreCurr,u8_DIDSta_TurnLampRRThreCurr,u8_TurnLampRRThreCurr,u8_DIDSta_TurnLampFLThreCurr,u8_TurnLampFLThreCurr,u8_DIDSta_TurnLampRLThreCurr,u8_TurnLampRLThreCurr,u8_DIDSta_FMHTimer,u8_FMHTimer,u8_DIDSta_AutoLock,u8_AutoLock,u8_DIDSta_DRLDis,u8_DRLDis,u8_DIDSta_USSConfig,u8Array16_USSConfig,u8_DIDSta_TireSize,u8Array16_TireSize,u8_DIDSta_APSFunConfig,u8Array16_APSFunConfig
  BHAL_DIDOrigOutput_raw8 : Outport
  wires:
  BHAL_DIDGetData_raw/1 -> [BHAL_DIDGetData_raw]
  VHAL_DIDFlashXWDMode_raw8/1 -> [VHAL_DIDFlashXWDMode_raw8]
  VHAL_DIDFlashDKCKey_raw8/1 -> [VHAL_DIDFlashDKCKey_raw8]
  VHAL_DIDFlashDynoMode_raw8/1 -> [VHAL_DIDFlashDynoMode_raw8]
  VHAL_DIDFlashTurnLampFRThreCurr_raw8/1 -> [VHAL_DIDFlashTurnLampFRThreCurr_raw8]
  VHAL_DIDFlashTurnLampRRThreCurr_raw8/1 -> [VHAL_DIDFlashTurnLampRRThreCurr_raw8]
  VHAL_DIDFlashTurnLampFLThreCurr_raw8/1 -> [VHAL_DIDFlashTurnLampFLThreCurr_raw8]
  VHAL_DIDFlashTurnLampRLThreCurr_raw8/1 -> [VHAL_DIDFlashTurnLampRLThreCurr_raw8]
  VHAL_DIDFlashFMHTimer_raw8/1 -> [VHAL_DIDFlashFMHTimer_raw8]
  VHAL_DIDFlashAutoLock_raw8/1 -> [VHAL_DIDFlashAutoLock_raw8]
  VHAL_DIDFlashDRLDis_raw8/1 -> [VHAL_DIDFlashDRLDis_raw8]
  VHAL_DIDFlashUSSConfig_raw8/1 -> [VHAL_DIDFlashUSSConfig_raw8]
  VHAL_DIDFlashTireSize_raw8/1 -> [VHAL_DIDFlashTireSize_raw8]
  VHAL_DIDFlashAPSFunConfig_raw8/1 -> [VHAL_DIDFlashAPSFunConfig_raw8]
  [BHAL_DIDGetData_raw] -> bus_selector/1
  bus_selector/1 -> UnitConverter/1  "<u8_DIDSta_XWDMode>"
  UnitConverter/1 -> [VHAL_DIDStaXWDMode_raw]  "VHAL_DIDStaXWDMode_raw"
  bus_selector/2 -> UnitConverter1/1  "<u8_XWDMode>"
  UnitConverter1/1 -> [VHAL_XWDMode_raw]  "VHAL_XWDMode_raw"
  bus_selector/3 -> UnitConverter2/1  "<u8_DIDSta_DKCKey>"
  UnitConverter2/1 -> [VHAL_DIDStaDKCKey_raw]  "VHAL_DIDStaDKCKey_raw"
  bus_selector/4 -> UnitConverter3/1  "<u8Array8_DKCKey>"
  UnitConverter3/1 -> [VHAL_DKCKey_raw]  "VHAL_DKCKey_raw"
  bus_selector/5 -> UnitConverter4/1  "<u8_DIDSta_DynoMode>"
  UnitConverter4/1 -> [VHAL_DIDStaDynoMode_raw]  "VHAL_DIDStaDynoMode_raw"
  bus_selector/6 -> UnitConverter5/1  "<u8_DynoMode>"
  UnitConverter5/1 -> [VHAL_DynoMode_raw]  "VHAL_DynoMode_raw"
  bus_selector/7 -> UnitConverter6/1  "<u8_DIDSta_TurnLampFRThreCurr>"
  UnitConverter6/1 -> [VHAL_DIDStaTurnLampFRThreCurr_raw]  "VHAL_DIDStaTurnLampFRThreCurr_raw"
  bus_selector/8 -> UnitConverter7/1  "<u8_TurnLampFRThreCurr>"
  UnitConverter7/1 -> [VHAL_TurnLampFRThreCurr_raw]  "VHAL_TurnLampFRThreCurr_raw"
  bus_selector/9 -> UnitConverter8/1  "<u8_DIDSta_TurnLampRRThreCurr>"
  UnitConverter8/1 -> [VHAL_DIDStaTurnLampRRThreCurr_raw]  "VHAL_DIDStaTurnLampRRThreCurr_raw"
  bus_selector/10 -> UnitConverter9/1  "<u8_TurnLampRRThreCurr>"
  UnitConverter9/1 -> [VHAL_TurnLampRRThreCurr_raw]  "VHAL_TurnLampRRThreCurr_raw"
  bus_selector/11 -> UnitConverter10/1  "<u8_DIDSta_TurnLampFLThreCurr>"
  UnitConverter10/1 -> [VHAL_DIDStaTurnLampFLThreCurr_raw]  "VHAL_DIDStaTurnLampFLThreCurr_raw"
  bus_selector/12 -> UnitConverter11/1  "<u8_TurnLampFLThreCurr>"
  UnitConverter11/1 -> [VHAL_TurnLampFLThreCurr_raw]  "VHAL_TurnLampFLThreCurr_raw"
  bus_selector/13 -> UnitConverter12/1  "<u8_DIDSta_TurnLampRLThreCurr>"
  UnitConverter12/1 -> [VHAL_DIDStaTurnLampRLThreCurr_raw]  "VHAL_DIDStaTurnLampRLThreCurr_raw"
  bus_selector/14 -> UnitConverter13/1  "<u8_TurnLampRLThreCurr>"
  UnitConverter13/1 -> [VHAL_TurnLampRLThreCurr_raw]  "VHAL_TurnLampRLThreCurr_raw"
  bus_selector/15 -> UnitConverter14/1  "<u8_DIDSta_FMHTimer>"
  UnitConverter14/1 -> [VHAL_DIDStaFMHTimer_raw]  "VHAL_DIDStaFMHTimer_raw"
  bus_selector/16 -> UnitConverter15/1  "<u8_FMHTimer>"
  UnitConverter15/1 -> [VHAL_FMHTimer_raw]  "VHAL_FMHTimer_raw"
  bus_selector/17 -> UnitConverter16/1  "<u8_DIDSta_AutoLock>"
  UnitConverter16/1 -> [VHAL_DIDStaAutoLock_raw]  "VHAL_DIDStaAutoLock_raw"
  bus_selector/18 -> UnitConverter17/1  "<u8_AutoLock>"
  UnitConverter17/1 -> [VHAL_AutoLock_raw]  "VHAL_AutoLock_raw"
  bus_selector/19 -> UnitConverter18/1  "<u8_DIDSta_DRLDis>"
  UnitConverter18/1 -> [VHAL_DIDStaDRLDis_raw]  "VHAL_DIDStaDRLDis_raw"
  bus_selector/20 -> UnitConverter19/1  "<u8_DRLDis>"
  UnitConverter19/1 -> [VHAL_DRLDis_raw]  "VHAL_DRLDis_raw"
  bus_selector/21 -> UnitConverter20/1  "<u8_DIDSta_USSConfig>"
  UnitConverter20/1 -> [VHAL_DIDStaUSSConfig_raw]  "VHAL_DIDStaUSSConfig_raw"
  bus_selector/22 -> UnitConverter21/1  "<u8Array16_USSConfig>"
  UnitConverter21/1 -> [VHAL_USSConfig_raw]  "VHAL_USSConfig_raw"
  bus_selector/23 -> UnitConverter22/1  "<u8_DIDSta_TireSize>"
  UnitConverter22/1 -> [VHAL_DIDStaTireSize_raw]  "VHAL_DIDStaTireSize_raw"
  bus_selector/24 -> UnitConverter23/1  "<u8Array16_TireSize>"
  UnitConverter23/1 -> [VHAL_TireSize_raw]  "VHAL_TireSize_raw"
  bus_selector/25 -> UnitConverter24/1  "<u8_DIDSta_APSFunConfig>"
  UnitConverter24/1 -> [VHAL_DIDStaAPSFunConfig_raw]  "VHAL_DIDStaAPSFunConfig_raw"
  bus_selector/26 -> UnitConverter25/1  "<u8Array16_APSFunConfig>"
  UnitConverter25/1 -> [VHAL_APSFunConfig_raw]  "VHAL_APSFunConfig_raw"
  [VHAL_XWDMode_raw] -> XWD switch/1
  [VHAL_DIDStaXWDMode_raw] -> XWD switch/2
  [VHAL_DIDFlashXWDMode_raw8] -> XWD switch/3
  XWD switch/1 -> [VHAL_DIDGetXWDMode_raw8]
  [VHAL_DKCKey_raw] -> WriteRandomNumberDKC/1
  [VHAL_DIDStaDKCKey_raw] -> WriteRandomNumberDKC/2
  [VHAL_DIDFlashDKCKey_raw8] -> WriteRandomNumberDKC/3
  WriteRandomNumberDKC/1 -> [VHAL_DIDGetDKCKey_raw8]
  [VHAL_DynoMode_raw] -> Dyno mode switch/1
  [VHAL_DIDStaDynoMode_raw] -> Dyno mode switch/2
  [VHAL_DIDFlashDynoMode_raw8] -> Dyno mode switch/3
  Dyno mode switch/1 -> [VHAL_DIDGetDynoMode_raw8]
  [VHAL_TurnLampFRThreCurr_raw] -> TurnLampFrontRightThresholdCurrent/1
  [VHAL_DIDStaTurnLampFRThreCurr_raw] -> TurnLampFrontRightThresholdCurrent/2
  [VHAL_DIDFlashTurnLampFRThreCurr_raw8] -> TurnLampFrontRightThresholdCurrent/3
  TurnLampFrontRightThresholdCurrent/1 -> [VHAL_DIDGetTurnLampFRThreCurr_raw8]
  [VHAL_TurnLampRRThreCurr_raw] -> TurnLampRearRightThresholdCurrent/1
  [VHAL_DIDStaTurnLampRRThreCurr_raw] -> TurnLampRearRightThresholdCurrent/2
  [VHAL_DIDFlashTurnLampRRThreCurr_raw8] -> TurnLampRearRightThresholdCurrent/3
  TurnLampRearRightThresholdCurrent/1 -> [VHAL_DIDGetTurnLampRRThreCurr_raw8]
  [VHAL_TurnLampFLThreCurr_raw] -> TurnLampFrontLeftThresholdCurrent/1
  [VHAL_DIDStaTurnLampFLThreCurr_raw] -> TurnLampFrontLeftThresholdCurrent/2
  [VHAL_DIDFlashTurnLampFLThreCurr_raw8] -> TurnLampFrontLeftThresholdCurrent/3
  TurnLampFrontLeftThresholdCurrent/1 -> [VHAL_DIDGetTurnLampFLThreCurr_raw8]
  [VHAL_TurnLampRLThreCurr_raw] -> TurnLampRearLeftThresholdCurrent/1
  [VHAL_DIDStaTurnLampRLThreCurr_raw] -> TurnLampRearLeftThresholdCurrent/2
  [VHAL_DIDFlashTurnLampRLThreCurr_raw8] -> TurnLampRearLeftThresholdCurrent/3
  TurnLampRearLeftThresholdCurrent/1 -> [VHAL_DIDGetTurnLampRLThreCurr_raw8]
  [VHAL_FMHTimer_raw] -> FollowMeHomeTimer/1
  [VHAL_DIDStaFMHTimer_raw] -> FollowMeHomeTimer/2
  [VHAL_DIDFlashFMHTimer_raw8] -> FollowMeHomeTimer/3
  FollowMeHomeTimer/1 -> [VHAL_DIDGetFMHTimer_raw8]
  [VHAL_AutoLock_raw] -> AutoLock/1
  [VHAL_DIDStaAutoLock_raw] -> AutoLock/2
  [VHAL_DIDFlashAutoLock_raw8] -> AutoLock/3
  AutoLock/1 -> [VHAL_DIDGetAutoLock_raw8]
  [VHAL_DRLDis_raw] -> DRLDisable/1
  [VHAL_DIDStaDRLDis_raw] -> DRLDisable/2
  [VHAL_DIDFlashDRLDis_raw8] -> DRLDisable/3
  DRLDisable/1 -> [VHAL_DIDGetDRLDis_raw8]
  [VHAL_USSConfig_raw] -> apsUssConfiguration/1
  [VHAL_DIDStaUSSConfig_raw] -> apsUssConfiguration/2
  [VHAL_DIDFlashUSSConfig_raw8] -> apsUssConfiguration/3
  apsUssConfiguration/1 -> [VHAL_DIDGetUSSConfig_raw8]
  [VHAL_TireSize_raw] -> apsVehicleTireSize/1
  [VHAL_DIDStaTireSize_raw] -> apsVehicleTireSize/2
  [VHAL_DIDFlashTireSize_raw8] -> apsVehicleTireSize/3
  apsVehicleTireSize/1 -> [VHAL_DIDGetTireSize_raw8]
  [VHAL_APSFunConfig_raw] -> apsFunctionConfiguration/1
  [VHAL_DIDStaAPSFunConfig_raw] -> apsFunctionConfiguration/2
  [VHAL_DIDFlashAPSFunConfig_raw8] -> apsFunctionConfiguration/3
  apsFunctionConfiguration/1 -> [VHAL_DIDGetAPSFunConfig_raw8]
  [VHAL_DIDGetXWDMode_raw8] -> bus_Creator/1  "VHAL_DIDGetXWDMode_raw8"
  [VHAL_DIDGetDKCKey_raw8] -> bus_Creator/2  "VHAL_DIDGetDKCKey_raw8"
  [VHAL_DIDGetDynoMode_raw8] -> bus_Creator/3  "VHAL_DIDGetDynoMode_raw8"
  [VHAL_DIDGetTurnLampFRThreCurr_raw8] -> bus_Creator/4  "VHAL_DIDGetTurnLampFRThreCurr_raw8"
  [VHAL_DIDGetTurnLampRRThreCurr_raw8] -> bus_Creator/5  "VHAL_DIDGetTurnLampRRThreCurr_raw8"
  [VHAL_DIDGetTurnLampFLThreCurr_raw8] -> bus_Creator/6  "VHAL_DIDGetTurnLampFLThreCurr_raw8"
  [VHAL_DIDGetTurnLampRLThreCurr_raw8] -> bus_Creator/7  "VHAL_DIDGetTurnLampRLThreCurr_raw8"
  [VHAL_DIDGetFMHTimer_raw8] -> bus_Creator/8  "VHAL_DIDGetFMHTimer_raw8"
  [VHAL_DIDGetAutoLock_raw8] -> bus_Creator/9  "VHAL_DIDGetAutoLock_raw8"
  [VHAL_DIDGetDRLDis_raw8] -> bus_Creator/10  "VHAL_DIDGetDRLDis_raw8"
  [VHAL_DIDGetUSSConfig_raw8] -> bus_Creator/11  "VHAL_DIDGetUSSConfig_raw8"
  [VHAL_DIDGetTireSize_raw8] -> bus_Creator/12  "VHAL_DIDGetTireSize_raw8"
  [VHAL_DIDGetAPSFunConfig_raw8] -> bus_Creator/13  "VHAL_DIDGetAPSFunConfig_raw8"
  bus_Creator/1 -> BHAL_DIDOrigOutput_raw8/1

== system SWC_FDC_type/run_SWC_FDC_RxTx_5ms_sys/Halin_CDD/Halin_SYS/FlashACForceOFF_Verify ==
  In1 : Inport
  Compare To Constant : simulink/Logic and Bit Operations/Compare To Constant  relop=>  const=1  OutDataTypeStr=boolean
  Compare To Constant1 : simulink/Logic and Bit Operations/Compare To Constant  relop=<  const=0  OutDataTypeStr=boolean
  Constant : Constant  Value=ZERO_INT
  Logical Operator : Logic  Operator=OR  AllPortsSameDT=off  OutDataTypeStr=boolean
  Switch : Switch  Criteria=u2 > Threshold
  Out1 : Outport
  wires:
  In1/1 -> Switch/3, Compare To Constant1/1, Compare To Constant/1
  Constant/1 -> Switch/1
  Switch/1 -> Out1/1
  Logical Operator/1 -> Switch/2
  Compare To Constant/1 -> Logical Operator/1
  Compare To Constant1/1 -> Logical Operator/2

== system SWC_FDC_type/run_SWC_FDC_RxTx_5ms_sys/Halin_CDD/Halin_SYS/FlashACModeMem_Verify ==
  In1 : Inport
  Compare To Constant : simulink/Logic and Bit Operations/Compare To Constant  relop=>  const=2  OutDataTypeStr=boolean
  Compare To Constant1 : simulink/Logic and Bit Operations/Compare To Constant  relop=<  const=0  OutDataTypeStr=boolean
  Constant : Constant  Value=ONE_INT
  Logical Operator : Logic  Operator=OR  AllPortsSameDT=off  OutDataTypeStr=boolean
  Switch : Switch  Criteria=u2 > Threshold
  Out1 : Outport
  wires:
  Compare To Constant1/1 -> Logical Operator/2
  Compare To Constant/1 -> Logical Operator/1
  Logical Operator/1 -> Switch/2
  Switch/1 -> Out1/1
  Constant/1 -> Switch/1
  In1/1 -> Compare To Constant/1, Compare To Constant1/1, Switch/3

== system SWC_FDC_type/run_SWC_FDC_RxTx_5ms_sys/Halin_CDD/Halin_SYS/FlashAPMDoorControlSta ==
  In1 : Inport
  Compare To Constant : simulink/Logic and Bit Operations/Compare To Constant  relop=>  const=1  OutDataTypeStr=boolean
  Compare To Constant1 : simulink/Logic and Bit Operations/Compare To Constant  relop=<  const=0  OutDataTypeStr=boolean
  Constant : Constant  Value=ONE_INT
  Logical Operator : Logic  Operator=OR  AllPortsSameDT=off  OutDataTypeStr=boolean
  Switch : Switch  Criteria=u2 > Threshold
  Out1 : Outport
  wires:
  In1/1 -> Switch/3, Compare To Constant1/1, Compare To Constant/1
  Constant/1 -> Switch/1
  Switch/1 -> Out1/1
  Logical Operator/1 -> Switch/2
  Compare To Constant/1 -> Logical Operator/1
  Compare To Constant1/1 -> Logical Operator/2

== system SWC_FDC_type/run_SWC_FDC_RxTx_5ms_sys/Halin_CDD/Halin_SYS/FlashAirIntenZone1M_Verify ==
  In1 : Inport
  Compare To Constant : simulink/Logic and Bit Operations/Compare To Constant  relop=>  const=15  OutDataTypeStr=boolean
  Compare To Constant1 : simulink/Logic and Bit Operations/Compare To Constant  relop=<  const=1  OutDataTypeStr=boolean
  Constant : Constant  Value=ONE_INT
  Logical Operator : Logic  Operator=OR  AllPortsSameDT=off  OutDataTypeStr=boolean
  Switch : Switch  Criteria=u2 > Threshold
  Out1 : Outport
  wires:
  Compare To Constant1/1 -> Logical Operator/2
  Compare To Constant/1 -> Logical Operator/1
  Logical Operator/1 -> Switch/2
  Switch/1 -> Out1/1
  Constant/1 -> Switch/1
  In1/1 -> Compare To Constant/1, Compare To Constant1/1, Switch/3

== system SWC_FDC_type/run_SWC_FDC_RxTx_5ms_sys/Halin_CDD/Halin_SYS/FlashCCUSyncSts_Verify ==
  In1 : Inport
  Compare To Constant : simulink/Logic and Bit Operations/Compare To Constant  relop=>  const=1  OutDataTypeStr=boolean
  Compare To Constant1 : simulink/Logic and Bit Operations/Compare To Constant  relop=<  const=0  OutDataTypeStr=boolean
  Constant : Constant  Value=ZERO_INT
  Logical Operator : Logic  Operator=OR  AllPortsSameDT=off  OutDataTypeStr=boolean
  Switch : Switch  Criteria=u2 > Threshold
  Out1 : Outport
  wires:
  Compare To Constant1/1 -> Logical Operator/2
  Compare To Constant/1 -> Logical Operator/1
  Logical Operator/1 -> Switch/2
  Switch/1 -> Out1/1
  Constant/1 -> Switch/1
  In1/1 -> Compare To Constant/1, Compare To Constant1/1, Switch/3

== system SWC_FDC_type/run_SWC_FDC_RxTx_5ms_sys/Halin_CDD/Halin_SYS/FlashCountAlarm_Verify ==
  In1 : Inport
  Compare To Constant : simulink/Logic and Bit Operations/Compare To Constant  relop=>  const=15  OutDataTypeStr=boolean
  Compare To Constant1 : simulink/Logic and Bit Operations/Compare To Constant  relop=<  const=0  OutDataTypeStr=boolean
  Constant : Constant  Value=ZERO_INT
  Logical Operator : Logic  Operator=OR  AllPortsSameDT=off  OutDataTypeStr=boolean
  Switch : Switch  Criteria=u2 > Threshold
  Out1 : Outport
  wires:
  In1/1 -> Switch/3, Compare To Constant1/1, Compare To Constant/1
  Constant/1 -> Switch/1
  Switch/1 -> Out1/1
  Logical Operator/1 -> Switch/2
  Compare To Constant/1 -> Logical Operator/1
  Compare To Constant1/1 -> Logical Operator/2

== system SWC_FDC_type/run_SWC_FDC_RxTx_5ms_sys/Halin_CDD/Halin_SYS/FlashFaceM_Verify ==
  In1 : Inport
  Compare To Constant : simulink/Logic and Bit Operations/Compare To Constant  relop=>  const=1  OutDataTypeStr=boolean
  Compare To Constant1 : simulink/Logic and Bit Operations/Compare To Constant  relop=<  const=0  OutDataTypeStr=boolean
  Constant : Constant  Value=ONE_INT
  Logical Operator : Logic  Operator=OR  AllPortsSameDT=off  OutDataTypeStr=boolean
  Switch : Switch  Criteria=u2 > Threshold
  Out1 : Outport
  wires:
  Compare To Constant1/1 -> Logical Operator/2
  Compare To Constant/1 -> Logical Operator/1
  Logical Operator/1 -> Switch/2
  Switch/1 -> Out1/1
  Constant/1 -> Switch/1
  In1/1 -> Compare To Constant/1, Compare To Constant1/1, Switch/3

== system SWC_FDC_type/run_SWC_FDC_RxTx_5ms_sys/Halin_CDD/Halin_SYS/FlashFace_Verify ==
  In1 : Inport
  Compare To Constant : simulink/Logic and Bit Operations/Compare To Constant  relop=>  const=1  OutDataTypeStr=boolean
  Compare To Constant1 : simulink/Logic and Bit Operations/Compare To Constant  relop=<  const=0  OutDataTypeStr=boolean
  Constant : Constant  Value=ONE_INT
  Logical Operator : Logic  Operator=OR  AllPortsSameDT=off  OutDataTypeStr=boolean
  Switch : Switch  Criteria=u2 > Threshold
  Out1 : Outport
  wires:
  In1/1 -> Compare To Constant/1, Compare To Constant1/1, Switch/3
  Constant/1 -> Switch/1
  Switch/1 -> Out1/1
  Logical Operator/1 -> Switch/2
  Compare To Constant/1 -> Logical Operator/1
  Compare To Constant1/1 -> Logical Operator/2

== system SWC_FDC_type/run_SWC_FDC_RxTx_5ms_sys/Halin_CDD/Halin_SYS/FlashFootM_Verify ==
  In1 : Inport
  Compare To Constant : simulink/Logic and Bit Operations/Compare To Constant  relop=>  const=1  OutDataTypeStr=boolean
  Compare To Constant1 : simulink/Logic and Bit Operations/Compare To Constant  relop=<  const=0  OutDataTypeStr=boolean
  Constant : Constant  Value=ZERO_INT
  Logical Operator : Logic  Operator=OR  AllPortsSameDT=off  OutDataTypeStr=boolean
  Switch : Switch  Criteria=u2 > Threshold
  Out1 : Outport
  wires:
  In1/1 -> Switch/3, Compare To Constant1/1, Compare To Constant/1
  Constant/1 -> Switch/1
  Switch/1 -> Out1/1
  Logical Operator/1 -> Switch/2
  Compare To Constant/1 -> Logical Operator/1
  Compare To Constant1/1 -> Logical Operator/2

== system SWC_FDC_type/run_SWC_FDC_RxTx_5ms_sys/Halin_CDD/Halin_SYS/FlashFoot_Verify ==
  In1 : Inport
  Compare To Constant : simulink/Logic and Bit Operations/Compare To Constant  relop=>  const=1  OutDataTypeStr=boolean
  Compare To Constant1 : simulink/Logic and Bit Operations/Compare To Constant  relop=<  const=0  OutDataTypeStr=boolean
  Constant : Constant  Value=ZERO_INT
  Logical Operator : Logic  Operator=OR  AllPortsSameDT=off  OutDataTypeStr=boolean
  Switch : Switch  Criteria=u2 > Threshold
  Out1 : Outport
  wires:
  Compare To Constant1/1 -> Logical Operator/2
  Compare To Constant/1 -> Logical Operator/1
  Logical Operator/1 -> Switch/2
  Switch/1 -> Out1/1
  Constant/1 -> Switch/1
  In1/1 -> Compare To Constant/1, Compare To Constant1/1, Switch/3

== system SWC_FDC_type/run_SWC_FDC_RxTx_5ms_sys/Halin_CDD/Halin_SYS/FlashFrost_Verify ==
  In1 : Inport
  Compare To Constant : simulink/Logic and Bit Operations/Compare To Constant  relop=>  const=1  OutDataTypeStr=boolean
  Compare To Constant1 : simulink/Logic and Bit Operations/Compare To Constant  relop=<  const=0  OutDataTypeStr=boolean
  Constant : Constant  Value=ZERO_INT
  Logical Operator : Logic  Operator=OR  AllPortsSameDT=off  OutDataTypeStr=boolean
  Switch : Switch  Criteria=u2 > Threshold
  Out1 : Outport
  wires:
  In1/1 -> Switch/3, Compare To Constant1/1, Compare To Constant/1
  Constant/1 -> Switch/1
  Switch/1 -> Out1/1
  Logical Operator/1 -> Switch/2
  Compare To Constant/1 -> Logical Operator/1
  Compare To Constant1/1 -> Logical Operator/2

== system SWC_FDC_type/run_SWC_FDC_RxTx_5ms_sys/Halin_CDD/Halin_SYS/FlashFuelDoorPos_Verify ==
  In1 : Inport
  Compare To Constant : simulink/Logic and Bit Operations/Compare To Constant  relop=>  const=1  OutDataTypeStr=boolean
  Compare To Constant1 : simulink/Logic and Bit Operations/Compare To Constant  relop=<  const=0  OutDataTypeStr=boolean
  Constant : Constant  Value=ZERO_INT
  Logical Operator : Logic  Operator=OR  AllPortsSameDT=off  OutDataTypeStr=boolean
  Switch : Switch  Criteria=u2 > Threshold
  Out1 : Outport
  wires:
  Compare To Constant1/1 -> Logical Operator/2
  Compare To Constant/1 -> Logical Operator/1
  Logical Operator/1 -> Switch/2
  Switch/1 -> Out1/1
  Constant/1 -> Switch/1
  In1/1 -> Compare To Constant/1, Compare To Constant1/1, Switch/3

== system SWC_FDC_type/run_SWC_FDC_RxTx_5ms_sys/Halin_CDD/Halin_SYS/FlashIVIPTGUSStaSW_Verify ==
  In1 : Inport
  Compare To Constant : simulink/Logic and Bit Operations/Compare To Constant  relop=>  const=1  OutDataTypeStr=boolean
  Compare To Constant1 : simulink/Logic and Bit Operations/Compare To Constant  relop=<  const=0  OutDataTypeStr=boolean
  Constant : Constant  Value=ZERO_INT
  Logical Operator : Logic  Operator=OR  AllPortsSameDT=off  OutDataTypeStr=boolean
  Switch : Switch  Criteria=u2 > Threshold
  Out1 : Outport
  wires:
  In1/1 -> Switch/3, Compare To Constant1/1, Compare To Constant/1
  Constant/1 -> Switch/1
  Switch/1 -> Out1/1
  Logical Operator/1 -> Switch/2
  Compare To Constant/1 -> Logical Operator/1
  Compare To Constant1/1 -> Logical Operator/2

== system SWC_FDC_type/run_SWC_FDC_RxTx_5ms_sys/Halin_CDD/Halin_SYS/FlashLockSetting_Verify ==
  In1 : Inport
  Compare To Constant : simulink/Logic and Bit Operations/Compare To Constant  relop=>  const=1  OutDataTypeStr=boolean
  Compare To Constant1 : simulink/Logic and Bit Operations/Compare To Constant  relop=<  const=0  OutDataTypeStr=boolean
  Constant : Constant  Value=ZERO_INT
  Logical Operator : Logic  Operator=OR  AllPortsSameDT=off  OutDataTypeStr=boolean
  Switch : Switch  Criteria=u2 > Threshold
  Out1 : Outport
  wires:
  In1/1 -> Switch/3, Compare To Constant1/1, Compare To Constant/1
  Constant/1 -> Switch/1
  Switch/1 -> Out1/1
  Logical Operator/1 -> Switch/2
  Compare To Constant/1 -> Logical Operator/1
  Compare To Constant1/1 -> Logical Operator/2

== system SWC_FDC_type/run_SWC_FDC_RxTx_5ms_sys/Halin_CDD/Halin_SYS/FlashMFRDNBrightReq_Verify ==
  In1 : Inport
  Compare To Constant : simulink/Logic and Bit Operations/Compare To Constant  relop=>  const=127  OutDataTypeStr=boolean
  Compare To Constant1 : simulink/Logic and Bit Operations/Compare To Constant  relop=<  const=0  OutDataTypeStr=boolean
  Constant : Constant  Value=ZERO_INT
  Logical Operator : Logic  Operator=OR  AllPortsSameDT=off  OutDataTypeStr=boolean
  Switch : Switch  Criteria=u2 > Threshold
  Out1 : Outport
  wires:
  Compare To Constant1/1 -> Logical Operator/2
  Compare To Constant/1 -> Logical Operator/1
  Logical Operator/1 -> Switch/2
  Switch/1 -> Out1/1
  Constant/1 -> Switch/1
  In1/1 -> Compare To Constant/1, Compare To Constant1/1, Switch/3

== system SWC_FDC_type/run_SWC_FDC_RxTx_5ms_sys/Halin_CDD/Halin_SYS/FlashMFSWTri_Verify ==
  In1 : Inport
  Compare To Constant : simulink/Logic and Bit Operations/Compare To Constant  relop=>  const=1  OutDataTypeStr=boolean
  Compare To Constant1 : simulink/Logic and Bit Operations/Compare To Constant  relop=<  const=0  OutDataTypeStr=boolean
  Constant : Constant  Value=ZERO_INT
  Logical Operator : Logic  Operator=OR  AllPortsSameDT=off  OutDataTypeStr=boolean
  Switch : Switch  Criteria=u2 > Threshold
  Out1 : Outport
  wires:
  Compare To Constant1/1 -> Logical Operator/2
  Compare To Constant/1 -> Logical Operator/1
  Logical Operator/1 -> Switch/2
  Switch/1 -> Out1/1
  Constant/1 -> Switch/1
  In1/1 -> Compare To Constant/1, Compare To Constant1/1, Switch/3

== system SWC_FDC_type/run_SWC_FDC_RxTx_5ms_sys/Halin_CDD/Halin_SYS/FlashMirrorFlodPos_Verify ==
  In1 : Inport
  Compare To Constant : simulink/Logic and Bit Operations/Compare To Constant  relop=>  const=1  OutDataTypeStr=boolean
  Compare To Constant1 : simulink/Logic and Bit Operations/Compare To Constant  relop=<  const=0  OutDataTypeStr=boolean
  Constant : Constant  Value=ZERO_INT
  Logical Operator : Logic  Operator=OR  AllPortsSameDT=off  OutDataTypeStr=boolean
  Switch : Switch  Criteria=u2 > Threshold
  Out1 : Outport
  wires:
  In1/1 -> Switch/3, Compare To Constant1/1, Compare To Constant/1
  Constant/1 -> Switch/1
  Switch/1 -> Out1/1
  Logical Operator/1 -> Switch/2
  Compare To Constant/1 -> Logical Operator/1
  Compare To Constant1/1 -> Logical Operator/2

== system SWC_FDC_type/run_SWC_FDC_RxTx_5ms_sys/Halin_CDD/Halin_SYS/FlashRecAutoFlg_Verify ==
  In1 : Inport
  Compare To Constant : simulink/Logic and Bit Operations/Compare To Constant  relop=>  const=1  OutDataTypeStr=boolean
  Compare To Constant1 : simulink/Logic and Bit Operations/Compare To Constant  relop=<  const=0  OutDataTypeStr=boolean
  Constant : Constant  Value=ZERO_INT
  Logical Operator : Logic  Operator=OR  AllPortsSameDT=off  OutDataTypeStr=boolean
  Switch : Switch  Criteria=u2 > Threshold
  Out1 : Outport
  wires:
  In1/1 -> Switch/3, Compare To Constant1/1, Compare To Constant/1
  Constant/1 -> Switch/1
  Switch/1 -> Out1/1
  Logical Operator/1 -> Switch/2
  Compare To Constant/1 -> Logical Operator/1
  Compare To Constant1/1 -> Logical Operator/2
